simulink model "Pitch_control"  (R2015a)
settings: Solver=ode45  StartTime=0.0  StopTime=20  RelTol=1e-3
values from neighbouring files (symbols this model uses):
  Cq = getBlockValue(CL,'Cq0')    [Hinf.m]    (also in HinfNest.m = getBlockValue(InnerLoop,'Cq0'); HinfStruct.m = getBlockValue(T,'Cq0'); HinfStruct_Loop.m = getBlockValue(T,'Cq0'); HinfStruct_Sensitivity.m)
  Ctheta = getBlockValue(CL,'Ctheta0')    [Hinf.m]    (also in HinfStruct.m = getBlockValue(T,'Ctheta0'); HinfStruct_Loop.m = getBlockValue(T,'Ctheta0'); HinfStruct_Sensitivity.m; HinfStruct_Sensitivity_uncertainty.m)
libraries: simulink x2
settings Model: Creator=pela  LastModifiedBy=pela

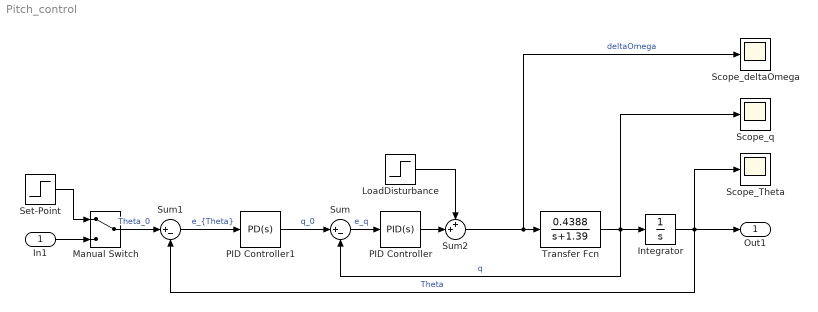
== system Pitch_control ==
  In1 : Inport
  Integrator : Integrator
  LoadDisturbance : Step  Time=5  After=-1  SampleTime=0
  Manual Switch : ManualSwitch
  PID Controller : simulink/Continuous/PID Controller  Controller=PID  TimeDomain=Continuous-time  SampleTime=-1  IntegratorMethod=Forward Euler  FilterMethod=Forward Euler  Form=Parallel  UseFilter=on  ControllerParametersSource=internal  P=Cq.Kp  I=Cq.Ki  D=Cq.Kd  N=100  InitialConditionSource=internal  InitialConditionForIntegrator=0  InitialConditionForFilter=0  ExternalReset=none  LimitOutput=off  UpperSaturationLimit=inf  LowerSaturationLimit=-inf  LinearizeAsGain=on  AntiWindupMode=none  Kb=1  TrackingMode=off  Kt=1  PParamMin=[]  PParamMax=[]  IParamMin=[]  IParamMax=[]  DParamMin=[]  DParamMax=[]  NParamMin=[]  NParamMax=[]  KbParamMin=[]  KbParamMax=[]  KtParamMin=[]  KtParamMax=[]  POutMin=[]  POutMax=[]  IOutMin=[]  IOutMax=[]  DOutMin=[]  DOutMax=[]  NOutMin=[]  NOutMax=[]  KbOutMin=[]  KbOutMax=[]  KtOutMin=[]  KtOutMax=[]  IntegratorOutMin=[]  IntegratorOutMax=[]  FilterOutMin=[]  FilterOutMax=[]  SumOutMin=[]  SumOutMax=[]  SumI1OutMin=[]  SumI1OutMax=[]  SumI2OutMin=[]  SumI2OutMax=[]  SumI3OutMin=[]  SumI3OutMax=[]  SumDOutMin=[]  SumDOutMax=[]  SaturationOutMin=[]  SaturationOutMax=[]  IntegratorContinuousStateAttributes=''  IntegratorStateMustResolveToSignalObject=off  IntegratorRTWStateStorageClass=Auto  FilterContinuousStateAttributes=''  FilterStateMustResolveToSignalObject=off  FilterRTWStateStorageClass=Auto  DifferentiatorICPrevScaledInput=0  DifferentiatorOutMin=[]  DifferentiatorOutMax=[]
  PID Controller1 : simulink/Continuous/PID Controller  Controller=PD  TimeDomain=Continuous-time  SampleTime=-1  IntegratorMethod=Forward Euler  FilterMethod=Forward Euler  Form=Parallel  UseFilter=on  ControllerParametersSource=internal  P=Ctheta.Kp  I=1  D=Ctheta.Kd  N=100  InitialConditionSource=internal  InitialConditionForIntegrator=0  InitialConditionForFilter=0  ExternalReset=none  LimitOutput=off  UpperSaturationLimit=inf  LowerSaturationLimit=-inf  LinearizeAsGain=on  AntiWindupMode=none  Kb=1  TrackingMode=off  Kt=1  PParamMin=[]  PParamMax=[]  IParamMin=[]  IParamMax=[]  DParamMin=[]  DParamMax=[]  NParamMin=[]  NParamMax=[]  KbParamMin=[]  KbParamMax=[]  KtParamMin=[]  KtParamMax=[]  POutMin=[]  POutMax=[]  IOutMin=[]  IOutMax=[]  DOutMin=[]  DOutMax=[]  NOutMin=[]  NOutMax=[]  KbOutMin=[]  KbOutMax=[]  KtOutMin=[]  KtOutMax=[]  IntegratorOutMin=[]  IntegratorOutMax=[]  FilterOutMin=[]  FilterOutMax=[]  SumOutMin=[]  SumOutMax=[]  SumI1OutMin=[]  SumI1OutMax=[]  SumI2OutMin=[]  SumI2OutMax=[]  SumI3OutMin=[]  SumI3OutMax=[]  SumDOutMin=[]  SumDOutMax=[]  SaturationOutMin=[]  SaturationOutMax=[]  IntegratorContinuousStateAttributes=''  IntegratorStateMustResolveToSignalObject=off  IntegratorRTWStateStorageClass=Auto  FilterContinuousStateAttributes=''  FilterStateMustResolveToSignalObject=off  FilterRTWStateStorageClass=Auto  DifferentiatorICPrevScaledInput=0  DifferentiatorOutMin=[]  DifferentiatorOutMax=[]
  Scope_Theta : Scope
  Scope_deltaOmega : Scope
      settings: SaveName=ScopeData2
  Scope_q : Scope
  Set-Point : Step  After=pi/12  SampleTime=0
  Sum : Sum  Inputs=|+-
  Sum1 : Sum  Inputs=|+-
  Sum2 : Sum  Inputs=++|
  Transfer Fcn : TransferFcn  Numerator=0.4388  Denominator=[1 1.39]
  Out1 : Outport
  wires:
  Sum/1 -> PID Controller/1  "e_q"
  Transfer Fcn/1 -> Scope_q/1, Sum/2, Integrator/1  "q"
  PID Controller1/1 -> Sum/1  "q_0"
  Sum1/1 -> PID Controller1/1  "e_{Theta}"
  Integrator/1 -> Scope_Theta/1, Out1/1, Sum1/2  "Theta"
  In1/1 -> Manual Switch/2
  Manual Switch/1 -> Sum1/1  "Theta_0"
  Set-Point/1 -> Manual Switch/1
  PID Controller/1 -> Sum2/2
  Sum2/1 -> Scope_deltaOmega/1, Transfer Fcn/1  "deltaOmega"
  LoadDisturbance/1 -> Sum2/1
